simulink model "reverb"  (R2025b)
settings: Solver=FixedStepDiscrete  StartTime=0.0  StopTime=inf  RelTol=1e-3
InitFcn:
  | Mix_rt=0.5;
  | RT60_rt=3;
  | Time1_rt=0.03;
  | Time2_rt=0.035;
  | Time3_rt=0.043;
  | Time4_rt=0.04;
model workspace (MATLAB code in the model file):
  | Gain_rt = Simulink.Parameter(1.0);
  | Bypass_rt = Simulink.Parameter(false);
  | Fs = 48000;
  | Ts = 1/Fs;
settings Model: Creator=linogarciamorales  LastModifiedBy=linogarciamorales
settings OptimizationCC: EnhancedBackFolding=on  PassReuseOutputArgsAs=Individual arguments  ZeroExternalMemoryAtStartup=off  ZeroInternalMemoryAtStartup=off  OptimizeBlockOrder=speed  DifferentSizesBufferReuse=on  OptimizationCustomize=off  EfficientTunableParamExpr=on
settings DebuggingCC: ParameterTunabilityLossMsg=error
settings SFSimCC: MATLABDynamicMemAlloc=off
settings RTWCC: SystemTargetFile=ert.tlc  GenCodeOnly=on  TemplateMakefile=ert_default_tmf  Description=Embedded Coder
settings CodeAppCC: ForceParamTrailComments=on  IgnoreCustomStorageClasses=off  OperatorAnnotations=on  SimulinkDataObjDesc=on  SFDataObjDesc=on  InsertBlockDesc=on
settings ERTTargetCC: InlinedParameterPlacement=Hierarchical  ERTCustomFileTemplate=example_file_process.tlc  TargetLangStandard=C99 (ISO)  GenerateSampleERTMain=on  SupportNonInlinedSFcns=on

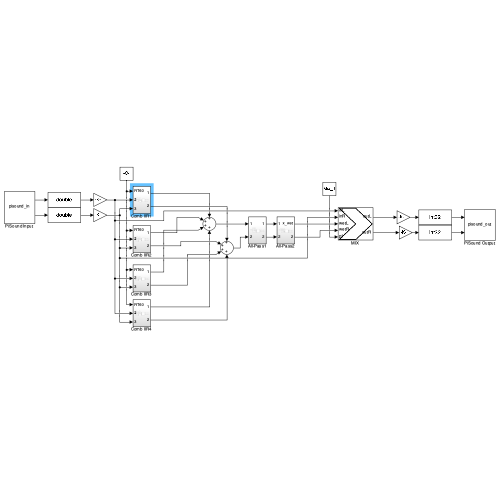
[thumbnail: Simulink's stored preview of the top-level diagram]
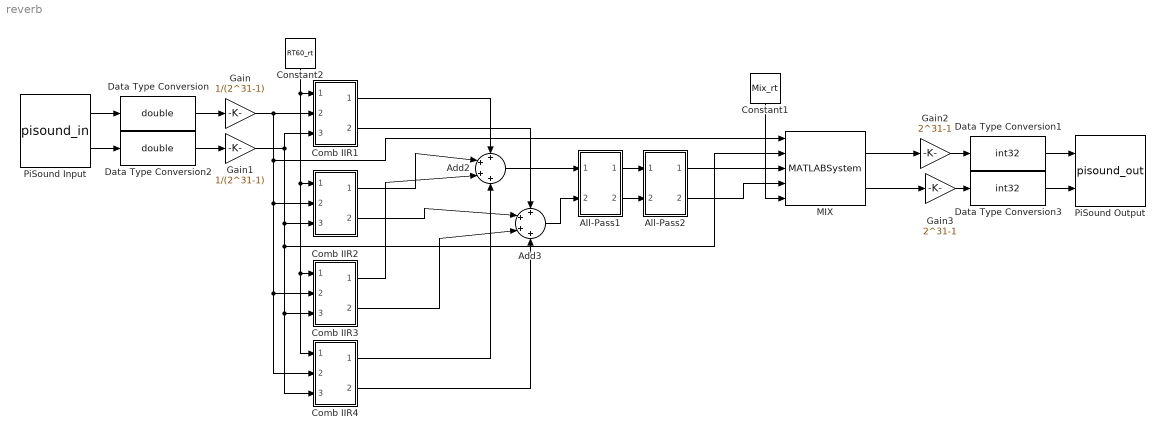
== system reverb ==
  Add2 : Sum  Inputs=++++  OutDataTypeStr=double  AccumDataTypeStr=double
  Add3 : Sum  Inputs=++++  OutDataTypeStr=double  AccumDataTypeStr=double
  All-Pass1 : Subsystem
  All-Pass2 : Subsystem
  Comb IIR1 : Subsystem
  Comb IIR2 : Subsystem
  Comb IIR3 : Subsystem
  Comb IIR4 : Subsystem
  Constant1 : Constant  Value=Mix_rt  OutDataTypeStr=double
  Constant2 : Constant  Value=RT60_rt  OutDataTypeStr=double
  Data Type Conversion : DataTypeConversion  OutDataTypeStr=double  SaturateOnIntegerOverflow=off  RndMeth=Floor
  Data Type Conversion1 : DataTypeConversion  OutDataTypeStr=int32  SaturateOnIntegerOverflow=off  RndMeth=Floor
  Data Type Conversion2 : DataTypeConversion  OutDataTypeStr=double  SaturateOnIntegerOverflow=off  RndMeth=Floor
  Data Type Conversion3 : DataTypeConversion  OutDataTypeStr=int32  SaturateOnIntegerOverflow=off  RndMeth=Floor
  Gain : Gain  Gain=1/(2^31-1)
  Gain1 : Gain  Gain=1/(2^31-1)
  Gain2 : Gain  Gain=2^31-1
  Gain3 : Gain  Gain=2^31-1
  MIX : MATLABSystem  System=mix_sys  N=128  Fs=48000  Mode=uint8( 0 )  SmoothTime=0.01  IndepInDB=false  SimulateUsing=Code generation
      mask Type: mix_sys
  PiSound Input : S-Function  FunctionName=pisound_in  Parameters=48000, 128, 0  SFunctionDeploymentMode=off  EnableBusSupport=off
  PiSound Output : S-Function  FunctionName=pisound_out  Parameters=48000, 128, 0  SFunctionDeploymentMode=off  EnableBusSupport=off
  wires:
  PiSound Input/1 -> Data Type Conversion/1
  PiSound Input/2 -> Data Type Conversion2/1
  Gain2/1 -> Data Type Conversion1/1
  Gain3/1 -> Data Type Conversion3/1
  Data Type Conversion/1 -> Gain/1
  Data Type Conversion2/1 -> Gain1/1
  All-Pass2/1(x_wet) -> MIX/3
  MIX/2 -> Gain3/1
  Gain1/1 -> Comb IIR2/3(In3), Comb IIR4/3(In3), Comb IIR3/3(In3), MIX/2, Comb IIR1/3(In3)
  Gain/1 -> MIX/1, Comb IIR2/2(In2), Comb IIR4/2(In2), Comb IIR3/2(In2), Comb IIR1/2(In2)
  Comb IIR2/1(Out1) -> Add2/2
  Comb IIR3/1(Out1) -> Add2/3
  Comb IIR4/1(Out1) -> Add2/4
  Comb IIR3/2(Out2) -> Add3/3
  Comb IIR4/2(Out2) -> Add3/4
  Comb IIR2/2(Out2) -> Add3/2
  All-Pass2/2(Out3) -> MIX/4
  Constant2/1 -> Comb IIR2/1(RT60), Comb IIR4/1(RT60), Comb IIR3/1(RT60), Comb IIR1/1(RT60)
  Comb IIR1/1(Out1) -> Add2/1
  Comb IIR1/2(Out2) -> Add3/1
  Add2/1 -> All-Pass1/1(In2)
  Add3/1 -> All-Pass1/2(In3)
  All-Pass1/1(Out1) -> All-Pass2/1(In2)
  All-Pass1/2(Out3) -> All-Pass2/2(In3)
  MIX/1 -> Gain2/1
  Constant1/1 -> MIX/5
  Data Type Conversion1/1 -> PiSound Output/1
  Data Type Conversion3/1 -> PiSound Output/2

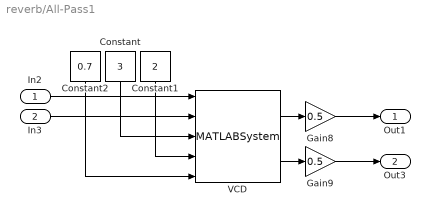
== system reverb/All-Pass1 ==
  In2 : Inport
  In3 : Inport  Port=2
  Constant : Constant  Value=3  OutDataTypeStr=uint8
  Constant1 : Constant  Value=2  OutDataTypeStr=double
  Constant2 : Constant  Value=0.7  OutDataTypeStr=double
  Gain8 : Gain  Gain=0.5  OutDataTypeStr=double
  Gain9 : Gain  Gain=0.5  OutDataTypeStr=double
  VCD : MATLABSystem  System=vcd_sys  N=128  Fs=48000  MaxDelay=2  Mode=uint8(1)  Delay=0.1  g=0.5  SimulateUsing=Code generation
      mask Type: vcd_sys
  Out1 : Outport
  Out3 : Outport  Port=2
  wires:
  Gain9/1 -> Out3/1
  In2/1 -> VCD/1
  Gain8/1 -> Out1/1
  Constant/1 -> VCD/3
  Constant2/1 -> VCD/5
  In3/1 -> VCD/2
  VCD/2 -> Gain9/1
  VCD/1 -> Gain8/1
  Constant1/1 -> VCD/4

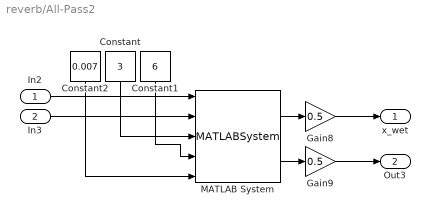
== system reverb/All-Pass2 ==
  In2 : Inport
  In3 : Inport  Port=2
  Constant : Constant  Value=3  OutDataTypeStr=uint8
  Constant1 : Constant  Value=6  OutDataTypeStr=double
  Constant2 : Constant  Value=0.007  OutDataTypeStr=double
  Gain8 : Gain  Gain=0.5  OutDataTypeStr=double
  Gain9 : Gain  Gain=0.5  OutDataTypeStr=double
  MATLAB System : MATLABSystem  System=vcd_sys  N=128  Fs=48000  MaxDelay=2  Mode=uint8(1)  Delay=0.1  g=0.5  SimulateUsing=Code generation
      mask Type: vcd_sys
  x_wet : Outport
  Out3 : Outport  Port=2
  wires:
  Gain9/1 -> Out3/1
  In2/1 -> MATLAB System/1
  Gain8/1 -> x_wet/1
  Constant/1 -> MATLAB System/3
  Constant2/1 -> MATLAB System/5
  In3/1 -> MATLAB System/2
  MATLAB System/2 -> Gain9/1
  MATLAB System/1 -> Gain8/1
  Constant1/1 -> MATLAB System/4

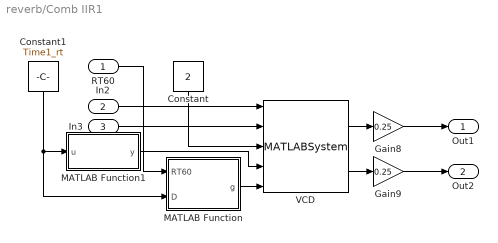
== system reverb/Comb IIR1 ==
  RT60 : Inport
  In2 : Inport  Port=2
  In3 : Inport  Port=3
  Constant : Constant  Value=2  OutDataTypeStr=uint8
  Constant1 : Constant  Value=Time1_rt  OutDataTypeStr=double
  Gain8 : Gain  Gain=0.25  OutDataTypeStr=double
  Gain9 : Gain  Gain=0.25  OutDataTypeStr=double
  MATLAB Function : MATLAB Function  TreatAsAtomicUnit=on
  MATLAB Function1 : MATLAB Function  TreatAsAtomicUnit=on
  VCD : MATLABSystem  System=vcd_sys  N=128  Fs=48000  MaxDelay=2  Mode=uint8(1)  Delay=0.1  g=0.5  SimulateUsing=Code generation
      mask Type: vcd_sys
  Out1 : Outport
  Out2 : Outport  Port=2
  wires:
  Gain9/1 -> Out2/1
  In2/1 -> VCD/1
  Gain8/1 -> Out1/1
  RT60/1 -> MATLAB Function/1(RT60)
  Constant/1 -> VCD/3
  MATLAB Function/1(g) -> VCD/5
  In3/1 -> VCD/2
  VCD/2 -> Gain9/1
  VCD/1 -> Gain8/1
  Constant1/1 -> MATLAB Function/2(D), MATLAB Function1/1(u)
  MATLAB Function1/1(y) -> VCD/4

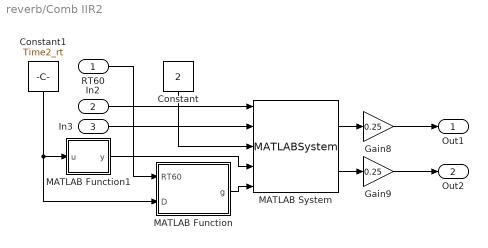
== system reverb/Comb IIR2 ==
  RT60 : Inport
  In2 : Inport  Port=2
  In3 : Inport  Port=3
  Constant : Constant  Value=2  OutDataTypeStr=uint8
  Constant1 : Constant  Value=Time2_rt  OutDataTypeStr=double
  Gain8 : Gain  Gain=0.25  OutDataTypeStr=double
  Gain9 : Gain  Gain=0.25  OutDataTypeStr=double
  MATLAB Function : MATLAB Function  TreatAsAtomicUnit=on
  MATLAB Function1 : MATLAB Function  TreatAsAtomicUnit=on
  MATLAB System : MATLABSystem  System=vcd_sys  N=128  Fs=48000  MaxDelay=2  Mode=uint8(1)  Delay=0.1  g=0.5  SimulateUsing=Code generation
      mask Type: vcd_sys
  Out1 : Outport
  Out2 : Outport  Port=2
  wires:
  Gain9/1 -> Out2/1
  In2/1 -> MATLAB System/1
  Gain8/1 -> Out1/1
  RT60/1 -> MATLAB Function/1(RT60)
  Constant/1 -> MATLAB System/3
  MATLAB Function/1(g) -> MATLAB System/5
  In3/1 -> MATLAB System/2
  MATLAB System/2 -> Gain9/1
  MATLAB System/1 -> Gain8/1
  Constant1/1 -> MATLAB Function/2(D), MATLAB Function1/1(u)
  MATLAB Function1/1(y) -> MATLAB System/4

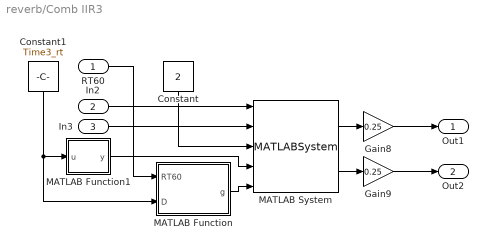
== system reverb/Comb IIR3 ==
  RT60 : Inport
  In2 : Inport  Port=2
  In3 : Inport  Port=3
  Constant : Constant  Value=2  OutDataTypeStr=uint8
  Constant1 : Constant  Value=Time3_rt  OutDataTypeStr=double
  Gain8 : Gain  Gain=0.25  OutDataTypeStr=double
  Gain9 : Gain  Gain=0.25  OutDataTypeStr=double
  MATLAB Function : MATLAB Function  TreatAsAtomicUnit=on
  MATLAB Function1 : MATLAB Function  TreatAsAtomicUnit=on
  MATLAB System : MATLABSystem  System=vcd_sys  N=128  Fs=48000  MaxDelay=2  Mode=uint8(1)  Delay=0.1  g=0.5  SimulateUsing=Code generation
      mask Type: vcd_sys
  Out1 : Outport
  Out2 : Outport  Port=2
  wires:
  Gain9/1 -> Out2/1
  In2/1 -> MATLAB System/1
  Gain8/1 -> Out1/1
  RT60/1 -> MATLAB Function/1(RT60)
  Constant/1 -> MATLAB System/3
  MATLAB Function/1(g) -> MATLAB System/5
  In3/1 -> MATLAB System/2
  MATLAB System/2 -> Gain9/1
  MATLAB System/1 -> Gain8/1
  Constant1/1 -> MATLAB Function/2(D), MATLAB Function1/1(u)
  MATLAB Function1/1(y) -> MATLAB System/4

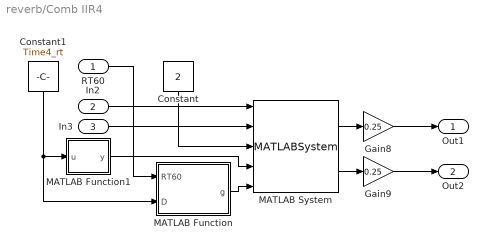
== system reverb/Comb IIR4 ==
  RT60 : Inport
  In2 : Inport  Port=2
  In3 : Inport  Port=3
  Constant : Constant  Value=2  OutDataTypeStr=uint8
  Constant1 : Constant  Value=Time4_rt  OutDataTypeStr=double
  Gain8 : Gain  Gain=0.25  OutDataTypeStr=double
  Gain9 : Gain  Gain=0.25  OutDataTypeStr=double
  MATLAB Function : MATLAB Function  TreatAsAtomicUnit=on
  MATLAB Function1 : MATLAB Function  TreatAsAtomicUnit=on
  MATLAB System : MATLABSystem  System=vcd_sys  N=128  Fs=48000  MaxDelay=2  Mode=uint8(1)  Delay=0.1  g=0.5  SimulateUsing=Code generation
      mask Type: vcd_sys
  Out1 : Outport
  Out2 : Outport  Port=2
  wires:
  Gain9/1 -> Out2/1
  In2/1 -> MATLAB System/1
  Gain8/1 -> Out1/1
  RT60/1 -> MATLAB Function/1(RT60)
  Constant/1 -> MATLAB System/3
  MATLAB Function/1(g) -> MATLAB System/5
  In3/1 -> MATLAB System/2
  MATLAB System/2 -> Gain9/1
  MATLAB System/1 -> Gain8/1
  Constant1/1 -> MATLAB Function/2(D), MATLAB Function1/1(u)
  MATLAB Function1/1(y) -> MATLAB System/4

== matlab function reverb/Comb IIR1/MATLAB Function ==
  data: RT60 input; g output; D input
function g = rt60_to_g(RT60, D)
%#codegen
% RT60: s (escalar)
% D   : s (escalar)

RT60min = 0.05;
if RT60 < RT60min
    RT60 = RT60min;
end

g = 10^(-3*D/RT60);

gmax = 0.95;
if g > gmax, g = gmax; end
if g < 0,    g = 0;    end
end

== matlab function reverb/Comb IIR4/MATLAB Function ==
  data: RT60 input; g output; D input
function g = rt60_to_g(RT60, D)
%#codegen
% RT60: s (escalar)
% D   : s (escalar)

RT60min = 0.05;
if RT60 < RT60min
    RT60 = RT60min;
end

g = 10^(-3*D/RT60);

gmax = 0.95;
if g > gmax, g = gmax; end
if g < 0,    g = 0;    end
end

== matlab function reverb/Comb IIR4/MATLAB Function1 ==
  data: u input; y output
function y = scalar2frame(u)
% u: escalar
% y: [N x 1]
N = 128;     % usa el mismo N del proyecto
y = u + zeros(N,1);
end

== matlab function reverb/Comb IIR1/MATLAB Function1 ==
  data: u input; y output
function y = scalar2frame(u)
% u: escalar
% y: [N x 1]
N = 128;     % usa el mismo N del proyecto
y = u + zeros(N,1);
end

== matlab function reverb/Comb IIR2/MATLAB Function ==
  data: RT60 input; g output; D input
function g = rt60_to_g(RT60, D)
%#codegen
% RT60: s (escalar)
% D   : s (escalar)

RT60min = 0.05;
if RT60 < RT60min
    RT60 = RT60min;
end

g = 10^(-3*D/RT60);

gmax = 0.95;
if g > gmax, g = gmax; end
if g < 0,    g = 0;    end
end

== matlab function reverb/Comb IIR2/MATLAB Function1 ==
  data: u input; y output
function y = scalar2frame(u)
% u: escalar
% y: [N x 1]
N = 128;     % usa el mismo N del proyecto
y = u + zeros(N,1);
end

== matlab function reverb/Comb IIR3/MATLAB Function1 ==
  data: u input; y output
function y = scalar2frame(u)
% u: escalar
% y: [N x 1]
N = 128;     % usa el mismo N del proyecto
y = u + zeros(N,1);
end

== matlab function reverb/Comb IIR3/MATLAB Function ==
  data: RT60 input; g output; D input
function g = rt60_to_g(RT60, D)
%#codegen
% RT60: s (escalar)
% D   : s (escalar)

RT60min = 0.05;
if RT60 < RT60min
    RT60 = RT60min;
end

g = 10^(-3*D/RT60);

gmax = 0.95;
if g > gmax, g = gmax; end
if g < 0,    g = 0;    end
end
